simulink model "Assignment_8"  (R2020b)
settings: Solver=VariableStepAuto  StartTime=0.0  StopTime=10.0  RelTol=1e-3
settings Model: Creator=Shantam Garg  LastModifiedBy=Shantam Garg

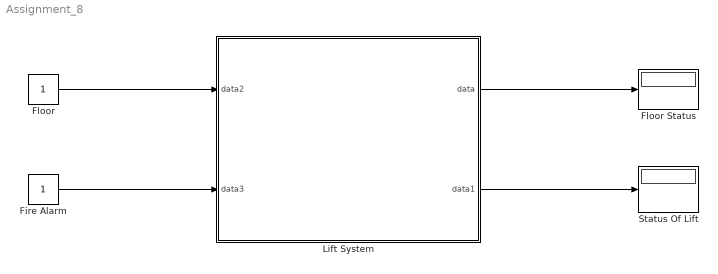
== system Assignment_8 ==
  Fire Alarm : Constant
  Floor : Constant
  Floor Status : Display
  Lift System : Stateflow chart  TreatAsAtomicUnit=on
  Status Of Lift : Display
  wires:
  Lift System/1(data) -> Floor Status/1
  Lift System/2(data1) -> Status Of Lift/1
  Floor/1 -> Lift System/1(data2)
  Fire Alarm/1 -> Lift System/2(data3)

== stateflow chart Assignment_8/Lift System ==
  state LiftOperation
    entry:
    status=0;
    state LiftOn
      state GroundFloor
        entry:
        status=1;
        during:
        Current=0;
        CheckFloor(Current);
        exit:
        status=0;
      state FirstFloor
        entry:
        status=1;
        during:
        Current=1;
        CheckFloor(Current);
        exit:
        status=0;
      state SecondFloor
        entry:
        status=1;
        during:
        Current=2;
        CheckFloor(Current);
        exit:
        status=0;
      state ThirdFloor
        entry:
        status=1;
        during:
        Current=3;
        CheckFloor(Current);
        exit:
        status=0;
      state FourthFloor
        entry:
        status=1
        during:
        Current=4;
        CheckFloor(Current);
        exit:
        status=0;
      state FifthFloor
        entry:
        status=1;
        during:
        Current=5;
        CheckFloor(Current);
        exit:
        status=0;
      (default) -> GroundFloor
      GroundFloor -> FirstFloor : up
      FirstFloor -> GroundFloor [order 2] : down
      FirstFloor -> SecondFloor [order 1] : up
      SecondFloor -> FirstFloor [order 2] : down
      SecondFloor -> ThirdFloor [order 1] : up
      ThirdFloor -> SecondFloor [order 2] : down
      ThirdFloor -> FourthFloor [order 1] : up
      FourthFloor -> ThirdFloor [order 1] : down
      FourthFloor -> FifthFloor [order 2] : up
      FifthFloor -> FourthFloor : down
    state LiftOff
      en:
      status=0;
      alarmStatus==0;
    (default) -> LiftOn
    LiftOff -> LiftOn : [fire==0]
    LiftOn -> LiftOff : [fire==1]
  data: data output; data1 output; data2 input; data3 input
